simulink library "GeminiRobotics"  (R2026a)
settings: Solver=VariableStepAuto
settings Model: Creator=smaddina  LastModifiedBy=smaddina

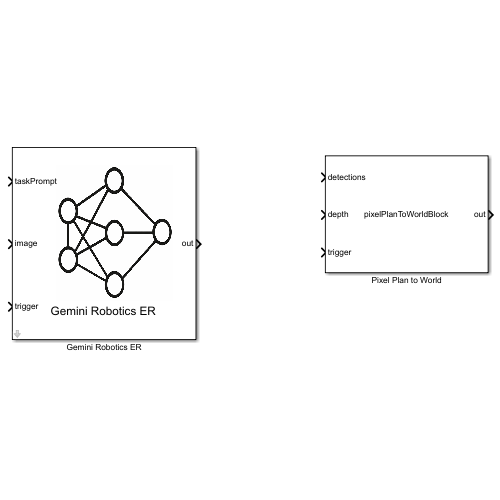
[thumbnail: Simulink's stored preview of the top-level diagram]
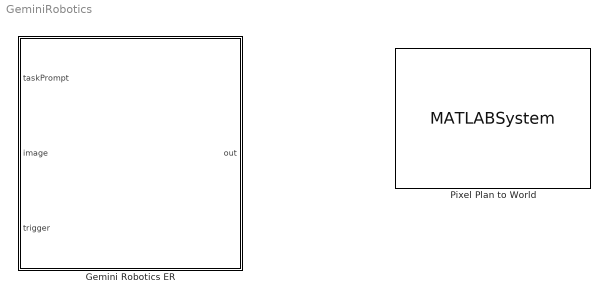
== system GeminiRobotics ==
  Gemini Robotics ER : Subsystem  mask{UseEnvApiKey=on, ApiKey=[], Mode=[], ScenarioPrompt=|, ThinkingBudget=0, SampleTime=inf}
      mask ScenarioPrompt=|
      | The scene is viewed from a camera mounted directly above the work cell, looking straight down.
      | The bin in the centre contains white plastic pipe fittings of four types: cross, tee, elbow, and straight.
      | Two placement tables are positioned on either side of the bin.
      mask prompts: UseEnvApiKey "Read API key from GEMINI_API_KEY env var"; ApiKey "API Key"; ScenarioPrompt "Scene context (prepended to every API call)"; ThinkingBudget "Thinking budget (0 = disabled, -1 = unlimited)"; SampleTime "Sample time"
      mask help: Calls the Gemini Robotics-ER 1.6 vision-language API with an image and task prompt. The API fires on the first simulation step and on each rising edge of the trigger input, and can also run periodically at a specified sample time. Results are cached between calls. Task-specific preprocessing and postprocessing are delegated to the Task object, making the block reusable for any Gemini-powered workflow such as object detection, task planning, or scene verification.
      mask init:
      | try
      |     set_param([gcb '/Sys'], 'UseEnvApiKey', UseEnvApiKey)
      |     set_param([gcb '/Sys'], 'ApiKey', ApiKey)
      |     set_param([gcb '/Sys'], 'Mode', Mode)
      |     set_param([gcb '/Sys'], 'ScenarioPrompt', ScenarioPrompt)
      |     set_param([gcb '/Sys'], 'ThinkingBudget', num2str(ThinkingBudget))
      | catch
      | end
      mask Display:
      | image(imread([fileparts(which('GeminiRobotics')) '/images/GeminiER.png']))
      | port_label('input',  1, 'taskPrompt')
      | port_label('input',  2, 'image')
      | port_label('input',  3, 'trigger')
      | port_label('output', 1, 'out')
      | text(0.5, 0.12, '\fontname{Arial}\fontsize{14}Gemini Robotics ER', 'HorizontalAlignment', 'center', 'VerticalAlignment', 'bottom', 'Interpreter', 'tex')
  Pixel Plan to World : MATLABSystem  System=pixelPlanToWorldBlock  FocalLength=750  PrincipalPoint=[640 360]  CameraLoc=[0.5 0 1.5]  CameraRot=pi/2*ones([1 3])  MaxBinDistance=0.95  DropHeightOffset=0.1  RobotOffsetZ=0.625001  MaxDetections=8
      mask Type: pixelPlanToWorldBlock

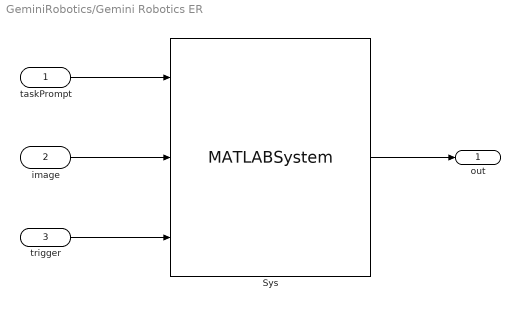
== system GeminiRobotics/Gemini Robotics ER ==
  taskPrompt : Inport
  image : Inport  Port=2
  trigger : Inport  Port=3
  Sys : MATLABSystem  System=geminiERBlock  UseEnvApiKey=on  ApiKey=[]  Mode=Mode  ScenarioPrompt=|  ThinkingBudget=0
      | The scene is viewed from a camera mounted directly above the work cell, looking straight down.
      | The bin in the centre contains white plastic pipe fittings of four types: cross, tee, elbow, and straight.
      | Two placement tables are positioned on either side of the bin.
      mask Type: geminiERBlock
  out : Outport
  wires:
  taskPrompt/1 -> Sys/1
  image/1 -> Sys/2
  trigger/1 -> Sys/3
  Sys/1 -> out/1
